simulink model "hodgkin_huxley_model"  (R2019b)
settings: Solver=VariableStepAuto  StartTime=0.0  StopTime=60  RelTol=1e-3
undefined symbols (not defined in the file or in its folder): Cm, g_K, g_L, g_Na, V_K, V_L, V_Na, V_r
settings Model: Creator=User  LastModifiedBy=User

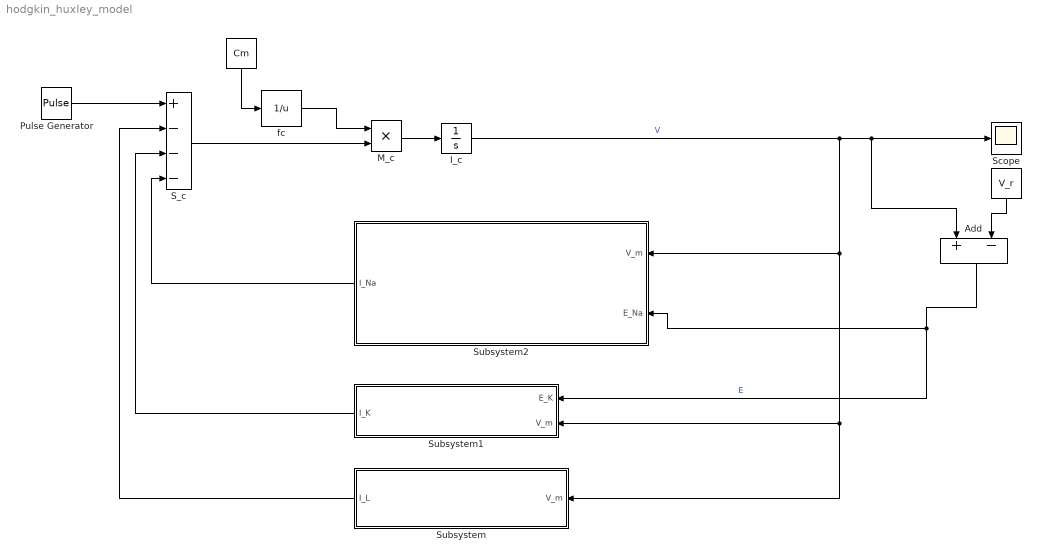
== system hodgkin_huxley_model ==
  "   " : Constant  Value=Cm
  "     " : Constant  Value=V_r
  Add : Sum  Inputs=+-
  "I_c " : Integrator
  M_c : Product
  Pulse Generator : DiscretePulseGenerator  PulseType=Time based  Amplitude=60  Period=60  PulseWidth=5
  S_c : Sum  Inputs=+---
  Scope : Scope
  Subsystem : Subsystem
  Subsystem1 : Subsystem
  Subsystem2 : Subsystem
  fc : Fcn  Expr=1/u
  wires:
  Pulse Generator/1 -> S_c/1
  "   "/1 -> fc/1
  S_c/1 -> M_c/2
  fc/1 -> M_c/1
  M_c/1 -> "I_c "/1
  "I_c "/1 -> Scope/1, Add/1, Subsystem/1(V_m), Subsystem1/2(V_m), Subsystem2/1(V_m)  "V"
  "     "/1 -> Add/2
  Add/1 -> Subsystem2/2(E_Na), Subsystem1/1(E_K)  "E"
  Subsystem/1(I_L) -> S_c/2
  Subsystem1/1(I_K) -> S_c/3
  Subsystem2/1(I_Na) -> S_c/4

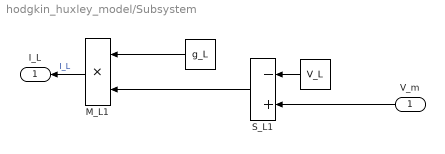
== system hodgkin_huxley_model/Subsystem ==
  V_m : Inport
  "     " : Constant  Value=V_L
  "            " : Constant  Value=g_L
  M_L1 : Product
  "S_L1 " : Sum  Inputs=-+
  I_L : Outport
  wires:
  "S_L1 "/1 -> M_L1/2
  M_L1/1 -> I_L/1  "I_L"
  "     "/1 -> "S_L1 "/1
  "            "/1 -> M_L1/1
  V_m/1 -> "S_L1 "/2

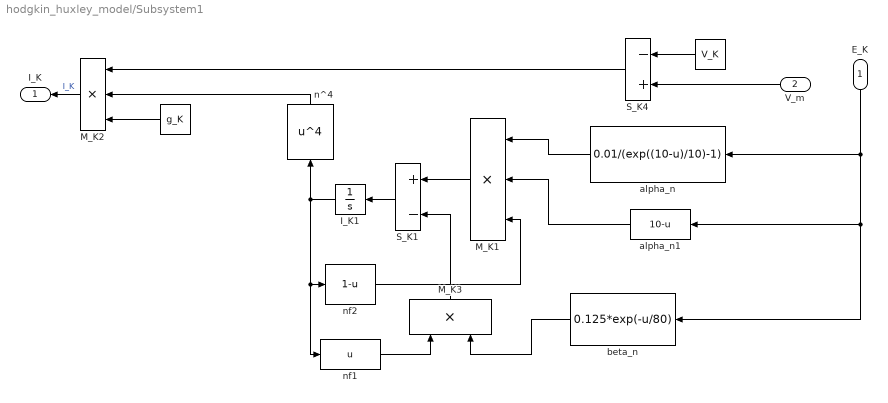
== system hodgkin_huxley_model/Subsystem1 ==
  E_K : Inport
  V_m : Inport  Port=2
  " " : Constant  Value=V_K
  "      " : Constant  Value=g_K
  I_K1 : Integrator
  M_K1 : Product  Inputs=3
  M_K2 : Product  Inputs=3
  M_K3 : Product
  S_K1 : Sum  Inputs=+-
  S_K4 : Sum  Inputs=-+
  alpha_n : Fcn  Expr=0.01/(exp((10-u)/10)-1)
  alpha_n1 : Fcn  Expr=10-u
  beta_n : Fcn  Expr=0.125*exp(-u/80)
  n^4 : Fcn  Expr=u^4
  "nf1 " : Fcn  Expr=u
  nf2 : Fcn  Expr=1-u
  I_K : Outport
  wires:
  M_K3/1 -> S_K1/2
  E_K/1 -> alpha_n1/1, beta_n/1, alpha_n/1
  I_K1/1 -> "nf1 "/1, nf2/1, n^4/1
  M_K1/1 -> S_K1/1
  " "/1 -> S_K4/1
  S_K4/1 -> M_K2/1
  S_K1/1 -> I_K1/1
  alpha_n/1 -> M_K1/1
  V_m/1 -> S_K4/2
  "      "/1 -> M_K2/3
  n^4/1 -> M_K2/2
  beta_n/1 -> M_K3/2
  M_K2/1 -> I_K/1  "I_K"
  "nf1 "/1 -> M_K3/1
  alpha_n1/1 -> M_K1/2
  nf2/1 -> M_K1/3

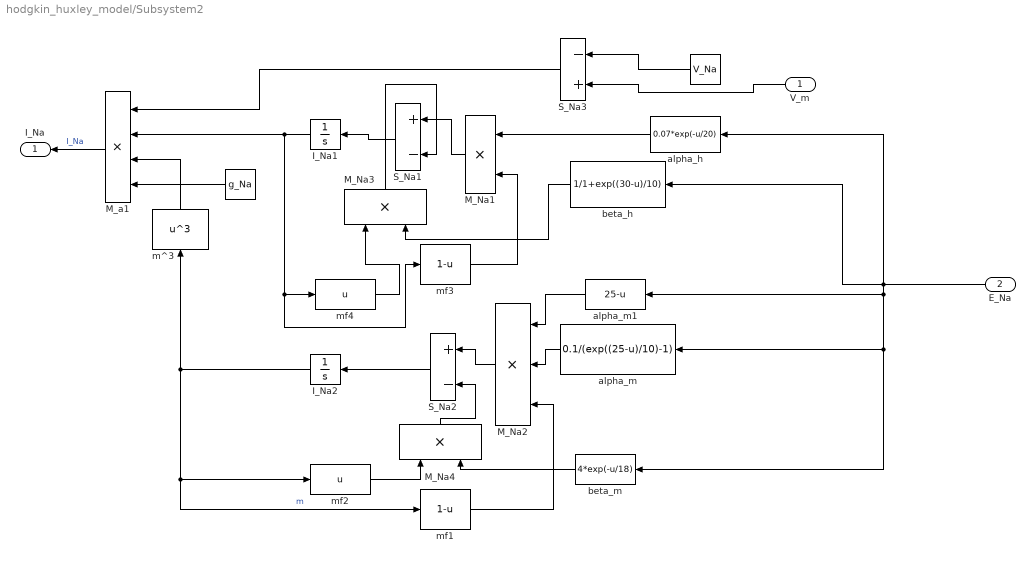
== system hodgkin_huxley_model/Subsystem2 ==
  V_m : Inport
  E_Na : Inport  Port=2
  " " : Constant  Value=g_Na
  "  " : Constant  Value=V_Na
  I_Na1 : Integrator
  I_Na2 : Integrator
  M_Na1 : Product
  M_Na2 : Product  Inputs=3
  M_Na3 : Product
  M_Na4 : Product
  "M_a1 " : Product  Inputs=4
  S_Na1 : Sum  Inputs=+-
  S_Na2 : Sum  Inputs=+-
  "S_Na3 " : Sum  Inputs=-+
  alpha_h : Fcn  Expr=0.07*exp(-u/20)
  alpha_m : Fcn  Expr=0.1/(exp((25-u)/10)-1)
  alpha_m1 : Fcn  Expr=25-u
  beta_h : Fcn  Expr=1/1+exp((30-u)/10)
  beta_m : Fcn  Expr=4*exp(-u/18)
  "m^3 " : Fcn  Expr=u^3
  mf1 : Fcn  Expr=1-u
  mf2 : Fcn  Expr=u
  mf3 : Fcn  Expr=1-u
  mf4 : Fcn  Expr=u
  I_Na : Outport
  wires:
  " "/1 -> "M_a1 "/4
  M_Na4/1 -> S_Na2/2
  I_Na1/1 -> "M_a1 "/2, mf3/1, mf4/1
  mf3/1 -> M_Na1/2
  alpha_h/1 -> M_Na1/1
  I_Na2/1 -> "m^3 "/1, mf1/1, mf2/1  "m"
  "  "/1 -> "S_Na3 "/1
  alpha_m1/1 -> M_Na2/1
  alpha_m/1 -> M_Na2/2
  mf1/1 -> M_Na2/3
  "m^3 "/1 -> "M_a1 "/3
  beta_m/1 -> M_Na4/2
  M_Na2/1 -> S_Na2/1
  mf2/1 -> M_Na4/1
  mf4/1 -> M_Na3/1
  S_Na2/1 -> I_Na2/1
  "S_Na3 "/1 -> "M_a1 "/1
  S_Na1/1 -> I_Na1/1
  beta_h/1 -> M_Na3/2
  M_Na3/1 -> S_Na1/2
  M_Na1/1 -> S_Na1/1
  V_m/1 -> "S_Na3 "/2
  E_Na/1 -> beta_m/1, alpha_m/1, alpha_m1/1, beta_h/1, alpha_h/1
  "M_a1 "/1 -> I_Na/1  "I_Na"
